simulink model "lab3"  (R2012b)
settings: Solver=ode45  StartTime=0.0  StopTime=10.0  RelTol=1e-3
settings Model: Creator=student  LastModifiedBy=student

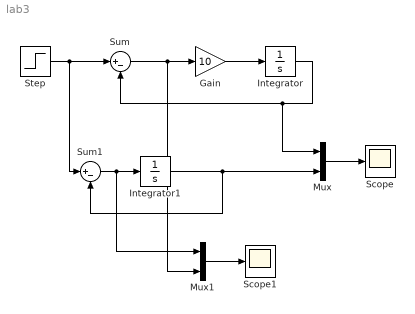
== system lab3 ==
  Gain : Gain  Gain=10
  Integrator : Integrator
  Integrator1 : Integrator
  Mux : Mux  Inputs=2
  Mux1 : Mux  Inputs=2
  Scope : Scope
  Scope1 : Scope
  Step : Step  Time=0  SampleTime=0
  Sum : Sum  Inputs=|+-
  Sum1 : Sum  Inputs=|+-
  wires:
  Integrator/1 -> Mux/1, Sum/2
  Step/1 -> Sum1/1, Sum/1
  Sum/1 -> Mux1/2, Gain/1
  Gain/1 -> Integrator/1
  Sum1/1 -> Mux1/1, Integrator1/1
  Mux/1 -> Scope/1
  Integrator1/1 -> Sum1/2, Mux/2
  Mux1/1 -> Scope1/1
